simulink model "test_SlungQuadDynamic"  (R2021a)
settings: Solver=VariableStepAuto  StartTime=0.0  StopTime=10.0  RelTol=1e-3
settings Model: Creator=Cindio  LastModifiedBy=Cindio

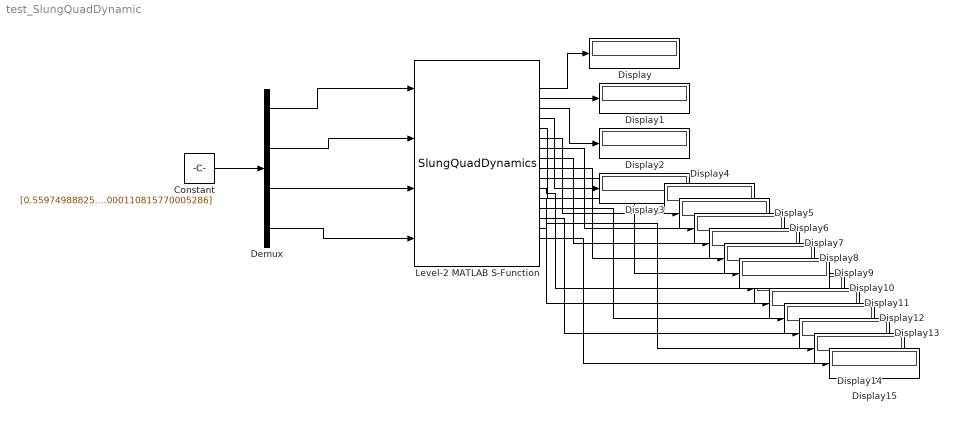
== system test_SlungQuadDynamic ==
  Constant : Constant  Value=[0.559749888250068,2.03629310837718,1.03864119408452,-0.000110815770005286]
  Demux : Demux
  Display{,1..15} (16 alike) : Display
  Level-2 MATLAB S-Function : M-S-Function  FunctionName=SlungQuadDynamics
  wires:
  Demux/1 -> Level-2 MATLAB S-Function/1
  Demux/2 -> Level-2 MATLAB S-Function/2
  Demux/3 -> Level-2 MATLAB S-Function/3
  Demux/4 -> Level-2 MATLAB S-Function/4
  Constant/1 -> Demux/1
  Level-2 MATLAB S-Function/1 -> Display/1
  Level-2 MATLAB S-Function/2 -> Display1/1
  Level-2 MATLAB S-Function/3 -> Display2/1
  Level-2 MATLAB S-Function/4 -> Display3/1
  Level-2 MATLAB S-Function/5 -> Display4/1
  Level-2 MATLAB S-Function/6 -> Display5/1
  Level-2 MATLAB S-Function/7 -> Display6/1
  Level-2 MATLAB S-Function/8 -> Display7/1
  Level-2 MATLAB S-Function/9 -> Display8/1
  Level-2 MATLAB S-Function/10 -> Display9/1
  Level-2 MATLAB S-Function/11 -> Display10/1
  Level-2 MATLAB S-Function/12 -> Display11/1
  Level-2 MATLAB S-Function/13 -> Display12/1
  Level-2 MATLAB S-Function/14 -> Display13/1
  Level-2 MATLAB S-Function/15 -> Display14/1
  Level-2 MATLAB S-Function/16 -> Display15/1
